simulink library "Lib_PF_BusLoadAC_TMATS"  (R2017a)
settings: Solver=ode45  StartTime=0.0  StopTime=10.0  RelTol=1e-3  EnableMultiTasking=on
Description:
  | Thomas Modules
settings Model: Creator=jwchapm2  LastModifiedBy=glthoma1
settings DataIOCC: LimitDataPoints=on  SaveFormat=Array
settings OptimizationCC: ExpressionDepthLimit=2147483647  LifeSpan=inf
settings DebuggingCC: UnderspecifiedInitializationDetection=Classic  MergeDetectMultiDrivingBlocksExec=none  SolverPrmCheckMsg=warning  StateNameClashWarn=warning  SFUnexpectedBacktrackingDiag=warning  SFNoUnconditionalDefaultTransitionDiag=warning  SFExecutionAtInitializationDiag=none
settings HardwareCC: ProdBitPerPointer=32  ProdBitPerSizeT=32  ProdBitPerPtrDiffT=32  ProdLargestAtomicFloat=None  ProdIntDivRoundTo=Undefined  ProdEndianess=Unspecified  ProdWordSize=32  ProdHWDeviceType=32-bit Generic
settings ModelReferenceCC: PropagateSignalLabelsOutOfModel=off
settings GRTTargetCC: TargetLangStandard=C89/C90 (ANSI)  GeneratePreprocessorConditionals=Disable all
settings ConfigComp: CovMetricSettings=dw  CovHtmlReporting=on  CovSaveCumulativeToWorkspaceVar=on  CovSaveSingleToWorkspaceVar=on  CovExternalEMLEnable=off

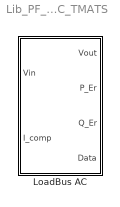
== system Lib_PF_BusLoadAC_TMATS ==
  LoadBus AC : Subsystem  mask{PeInEN_M=off, P_M=-4, QeInEN_M=off, Q_M=-2.5, BlkNm_M=double(gcb)}
      mask prompts: PeInEN_M "PeInEN_M - External Power Pelec"; BlkNm_M "Block name as double"
      mask init:
      | %Manage Reactive Power Inputs
      | if QeInEN_M == 1
      |     if strcmp(get_param([BlkNm_M '/Qelec'],'BlockType'),'Constant')
      |         MSK_ReplaceBlock_TMATS([BlkNm_M '/Qelec'],'built-in/Inport');
      |     end
      |     set_param([BlkNm_M '/Qelec'],'Port',num2str(2));
      | elseif QeInEN_M == 0
      |     if strcmp(get_param([BlkNm_M '/Qelec'],'BlockType'),'Inport')
      |         MSK_ReplaceBlock_TMATS([BlkNm_M '/Qelec'],'built-in/Constant');
      |         set_param([BlkNm_M '/Qelec'],'Value','Q_M');
      |     end
      | end
      | 
      | %Manage Power Inputs
      | if PeInEN_M == 1
      |     if strcmp(get_param([BlkNm_M '/Pelec'],'BlockType'),'Constant')
      |         MSK_ReplaceBlock_TMATS([BlkNm_M '/Pelec'],'built-in/Inport');
      |     end
      |     set_param([BlkNm_M '/Pelec'],'Port',num2str(2));
      | elseif PeInEN_M == 0
      |     if strcmp(get_param([BlkNm_M '/Pelec'],'BlockType'),'Inport')
      |         MSK_ReplaceBlock_TMATS([BlkNm_M '/Pelec'],'built-in/Constant');
      |         set_param([BlkNm_M '/Pelec'],'Value','P_M');
      |     end
      | end
      mask Callback PeInEN_M: MSK_SEC_Enables_TMATS('PeInEN_M',2,'dis')
      mask Callback QeInEN_M: MSK_SEC_Enables_TMATS('QeInEN_M',4,'dis')

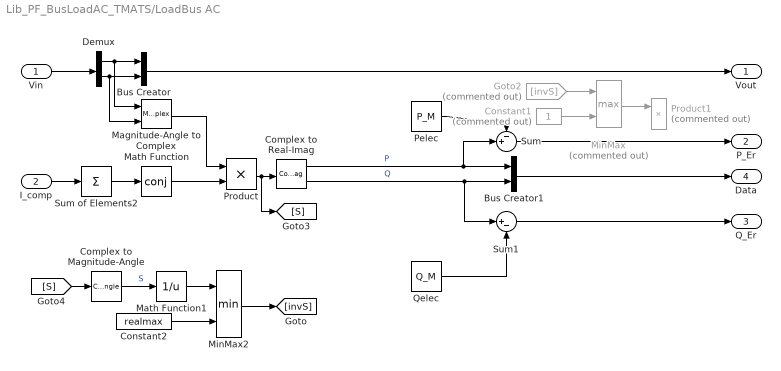
== system Lib_PF_BusLoadAC_TMATS/LoadBus AC ==
  Vin : Inport
  I_comp : Inport  Port=2
  Bus Creator : BusCreator  Inputs=2
  Bus Creator1 : BusCreator  Inputs=2
  Complex to Magnitude-Angle : ComplexToMagnitudeAngle  Output=Magnitude
  Complex to Real-Imag : ComplexToRealImag
  Constant1 : Constant  Commented=on
  Constant2 : Constant  Value=realmax
  Demux : Demux  Outputs=2
  Goto2 : From  Commented=on  GotoTag=invS
  Magnitude-Angle to Complex : MagnitudeAngleToComplex
  Math Function : Math  Operator=conj  SaturateOnIntegerOverflow=on
  Math Function1 : Math  Operator=reciprocal  SaturateOnIntegerOverflow=on
  MinMax : MinMax  Commented=on  Function=max  Inputs=2
  MinMax2 : MinMax  Inputs=2
  Pelec : Constant  Value=P_M
  Product : Product
  Product1 : Product  Commented=on
  Qelec : Constant  Value=Q_M
  Sum : Sum  Inputs=-+|
  Sum of Elements2 : Sum  Inputs=+
  Sum1 : Sum  Inputs=|+-
  Vout : Outport
  P_Er : Outport  Port=2
  Q_Er : Outport  Port=3
  Data : Outport  Port=4
  wires:
  I_comp/1 -> Sum of Elements2/1
  Product/1 -> [S], Complex to Real-Imag/1
  Math Function/1 -> Product/2
  Magnitude-Angle to Complex/1 -> Product/1
  Sum of Elements2/1 -> Math Function/1
  Complex to Real-Imag/1 -> Bus Creator1/1, Sum/2  "P"
  Pelec/1 -> Sum/1
  Qelec/1 -> Sum1/2
  Complex to Real-Imag/2 -> Bus Creator1/2, Sum1/1  "Q"
  Demux/2 -> Bus Creator/2, Magnitude-Angle to Complex/2
  Demux/1 -> Bus Creator/1, Magnitude-Angle to Complex/1
  Vin/1 -> Demux/1
  Bus Creator/1 -> Vout/1
  Complex to Magnitude-Angle/1 -> Math Function1/1  "S"
  [S] -> Complex to Magnitude-Angle/1
  Constant2/1 -> MinMax2/2
  Math Function1/1 -> MinMax2/1
  MinMax2/1 -> [invS]
  Constant1/1 -> MinMax/2
  Bus Creator1/1 -> Data/1
  MinMax/1 -> Product1/1
  Goto2/1 -> MinMax/1
  Sum1/1 -> Q_Er/1
  Sum/1 -> P_Er/1
